simulink model "Control_Logic_b_chk2"  (R2019b)
settings: Solver=VariableStepAuto  StartTime=Start_time  StopTime=Stop_time  RelTol=1e-3
values from neighbouring files (symbols this model uses):
  Aset_N1 = 2    [Parameter_control.m]
  Aset_N10 = -10    [Parameter_control.m]
  Aset_N11 = 10    [Parameter_control.m]
  Aset_N12 = 20    [Parameter_control.m]
  Aset_N2 = 30    [Parameter_control.m]
  Aset_N3 = 3    [Parameter_control.m]
  Aset_N4 = 5    [Parameter_control.m]
  Aset_N5 = 1    [Parameter_control.m]
  Aset_N6 = 0    [Parameter_control.m]
  Aset_N7 = 0.01    [Parameter_control.m]
  Aset_N8 = 2    [Parameter_control.m]
  Aset_N9 = 0.1    [Parameter_control.m]
  Dset_N1 = 1    [Parameter_control.m]
  Dset_N2 = 1    [Parameter_control.m]
  Sample_time = 0.1    [main.m]    (also in test_tool_initialize.m)
undefined symbols (not defined in the file or in its folder): DiscIntNeverNeededParam
(part 1 of 3)
settings Model: Creator=M156732  LastModifiedBy=yangy
settings DataIOCC: ReturnWorkspaceOutputs=off
settings DebuggingCC: ArithmeticOperatorsInVariantConditions=warning
settings ModelReferenceCC: ModelReferenceNumInstancesAllowed=Single
settings SFSimCC: CustomCodeUndefinedFunction=UseInterfaceOnly

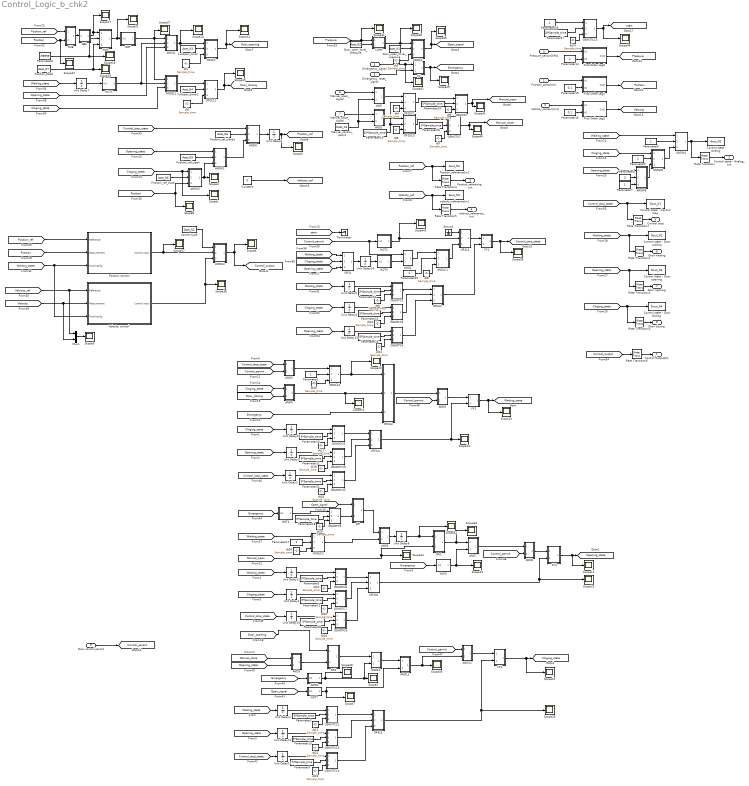
== system Control_Logic_b_chk2 ==
  Position_sensor[m] : Inport  OutDataTypeStr=double  Unit=mm  SampleTime=Sample_time
  Velocity_sensor[m/s] : Inport  Port=2  OutDataTypeStr=double  Unit=mm  SampleTime=Sample_time
  Pressure_sensor[kPa] : Inport  Port=3  OutDataTypeStr=double  Unit=kPa  SampleTime=Sample_time
  Emergency_signal : Inport  Port=4  OutDataTypeStr=boolean  SampleTime=Sample_time
  Emergency_reset_signal : Inport  Port=5  OutDataTypeStr=boolean  SampleTime=Sample_time
  Manual_open_signal : Inport  Port=6  OutDataTypeStr=boolean  SampleTime=Sample_time
  Manual_close_signal : Inport  Port=7  OutDataTypeStr=boolean  SampleTime=Sample_time
  Door control permit : Inport  Port=8  OutDataTypeStr=boolean  SampleTime=Sample_time
  ABS : Subsystem
  AND : Subsystem
  AND1 : Subsystem
  AND10 : Subsystem
  AND11 : Subsystem
  AND12 : Subsystem
  AND2 : Subsystem
  AND3 : Subsystem
  AND3L : Subsystem
  AND3L1 : Subsystem
  AND4 : Subsystem
  AND5 : Subsystem
  AND6 : Subsystem
  AND7 : Subsystem
  AND8 : Subsystem
  AND9 : Subsystem
  ANSW : Subsystem
  ANSW1 : Subsystem
  ANSW2 : Subsystem
  ANSW3 : Subsystem
  ANSW4 : Subsystem
  ANSW5 : Subsystem
  ANSW6 : Subsystem
  COMP : Subsystem
  Constant : Constant  Value=0
  Control state - Analog : ToWorkspace  VariableName=Aout_N2  SampleTime=Sample_time
  Control state - Control stop : ToWorkspace  VariableName=Dout_N1  SampleTime=Sample_time
  Control state - Door closing : ToWorkspace  VariableName=Dout_N4  SampleTime=Sample_time
  Control state - Door opening : ToWorkspace  VariableName=Dout_N3  SampleTime=Sample_time
  Control state - Door waiting : ToWorkspace  VariableName=Dout_N2  SampleTime=Sample_time
  Door_open_level_pressure : Constant  Value=Aset_N2  OutDataTypeStr=double  SampleTime=Sample_time
  Door_open_timer_pressure : Constant  Value=Aset_N1  OutDataTypeStr=double  SampleTime=Sample_time
  FF : Subsystem
  FF1 : Subsystem
  FF2 : Subsystem
  FF3 : Subsystem
  FF4 : Subsystem
  First Order Lag1 : Subsystem
  First Order Lag2 : Subsystem
  First Order Lag5 : Subsystem
  Fullopen_timer : Constant  Value=Aset_N3  OutDataTypeStr=double  SampleTime=Sample_time
  Fullopen_timer1 : Constant  Value=Aset_N4  OutDataTypeStr=double  SampleTime=Sample_time
  Ground : Ground
  HLM : Subsystem
  Manual_control_pemit : Constant  Value=Dset_N1  OutDataTypeStr=boolean  SampleTime=Sample_time
  Mux1 : Mux  Inputs=2
  NOT : Subsystem
  NOT1 : Subsystem
  NOT2 : Subsystem
  NOT3 : Subsystem
  NOT4 : Subsystem
  NOT5 : Subsystem
  NOT6 : Subsystem
  NOT7 : Subsystem
  OFDLC : Subsystem
  OFDLC1 : Subsystem
  OFDLC2 : Subsystem
  OFDLC3 : Subsystem
  ONDLC : Subsystem
  ONDLC1 : Subsystem
  ONDLC2 : Subsystem
  ONDLC3 : Subsystem
  OR : Subsystem
  OR1 : Subsystem
  OR2 : Subsystem
  OR3L : Subsystem
  OR3L1 : Subsystem
  OR3L2 : Subsystem
  OR3L3 : Subsystem
  OR3L4 : Subsystem
  OR3L5 : Subsystem
  OR3L6 : Subsystem
  OSHOTC : Subsystem
  OSHOTC1 : Subsystem
  OSHOTC10 : Subsystem
  OSHOTC11 : Subsystem
  OSHOTC12 : Subsystem
  OSHOTC13 : Subsystem
  OSHOTC14 : Subsystem
  OSHOTC15 : Subsystem
  OSHOTC2 : Subsystem
  OSHOTC3 : Subsystem
  OSHOTC4 : Subsystem
  OSHOTC5 : Subsystem
  OSHOTC6 : Subsystem
  OSHOTC7 : Subsystem
  OSHOTC8 : Subsystem
  OSHOTC9 : Subsystem
  Parameter{1,6..7,25} (4 alike) : Constant  OutDataTypeStr=int32  SampleTime=Sample_time
  Parameter{2..3,9..13,18,20..24,28..29} (15 alike) : Constant  Value=5*Sample_time  OutDataTypeStr=double  SampleTime=Sample_time
  Parameter14 : Constant  OutDataTypeStr=double  SampleTime=Sample_time
  Parameter15 : Constant  Value=0.1  OutDataTypeStr=double  SampleTime=Sample_time
  Parameter16 : Constant  Value=0.1  OutDataTypeStr=double  SampleTime=Sample_time
  Parameter17 : Constant  Value=2  OutDataTypeStr=int32  SampleTime=Sample_time
  Parameter19 : Constant  Value=10*Sample_time  OutDataTypeStr=double  SampleTime=Sample_time
  Parameter26 : Constant  OutDataTypeStr=boolean  SampleTime=Sample_time
  Parameter27 : Constant  Value=10*Sample_time  OutDataTypeStr=double  SampleTime=Sample_time
  Parameter4 : Constant  Value=3  OutDataTypeStr=int32  SampleTime=Sample_time
  Parameter5 : Constant  Value=2  OutDataTypeStr=int32  SampleTime=Sample_time
  Parameter8 : Constant  Value=-99999  OutDataTypeStr=double  SampleTime=Sample_time
  Position control : Subsystem
  Position_delta : Constant  Value=Aset_N7  OutDataTypeStr=double  SampleTime=Sample_time
  Position_ref_close : Constant  Value=Aset_N6  OutDataTypeStr=double  SampleTime=Sample_time
  Position_ref_close1 : Constant  Value=Aset_N6  OutDataTypeStr=double  SampleTime=Sample_time
  Position_ref_open : Constant  Value=Aset_N5  OutDataTypeStr=double  SampleTime=Sample_time
  Position_reference[m] : ToWorkspace  VariableName=Aout_N3  SampleTime=Sample_time
  Rate Transition{,1..7} (8 alike) : RateTransition  OutPortSampleTime=Sample_time
  SUB : Subsystem
  Scope{1..4,6..44} (43 alike) : Scope
  Terminator : Terminator
  Unit Delay{1..13,15..16} (15 alike) : UnitDelay  SampleTime=Sample_time  HasFrameUpgradeWarning=on
  Unit Delay14 : UnitDelay  InitialCondition=1  SampleTime=Sample_time  HasFrameUpgradeWarning=on
  Velocity control : Subsystem
  control type : Constant  Value=Dset_N2  OutDataTypeStr=boolean  SampleTime=Sample_time
  dt{1..12,14..19,21..24} (22 alike) : Constant  Value=Sample_time  OutDataTypeStr=double  SampleTime=Sample_time
  dt25 : Constant  Value=Sample_time  OutDataTypeStr=double
  dt26 : Constant  Value=Sample_time  OutDataTypeStr=double
  velocity_reference[m] : ToWorkspace  VariableName=Aout_N4  SampleTime=Sample_time
  Control Output[N] : Outport  OutDataTypeStr=double  Unit=N  SampleTime=Sample_time  VectorParamsAs1DForOutWhenUnconnected=off  LockScale=on
  Control state - Analog_out : Outport  Port=2  SampleTime=Sample_time  VectorParamsAs1DForOutWhenUnconnected=off
  Position_reference_out : Outport  Port=3  SampleTime=Sample_time  VectorParamsAs1DForOutWhenUnconnected=off
  velocity_reference_out : Outport  Port=4  SampleTime=Sample_time  VectorParamsAs1DForOutWhenUnconnected=off
  Control stop : Outport  Port=5  SampleTime=Sample_time  VectorParamsAs1DForOutWhenUnconnected=off
  Door waiting : Outport  Port=6  SampleTime=Sample_time  VectorParamsAs1DForOutWhenUnconnected=off
  Door opening : Outport  Port=7  SampleTime=Sample_time  VectorParamsAs1DForOutWhenUnconnected=off
  Door closing : Outport  Port=8  SampleTime=Sample_time  VectorParamsAs1DForOutWhenUnconnected=off
  tag scope: Cloging_state=global, Control_output=global, Control_permit=global, Control_stop_state=global, Door_closing=global, Door_opening=global, Emergency=global, Manual_close=global, Manual_open=global, Open_signal=global, Opening_state=global, Position=global, Position_ref=global, Pressure=global, Velocity=global, Velocity_ref=global, Waiting_state=global, start=global
  wires:
  FF2/1(Out1) -> Scope10/1, [Waiting_state]
  FF3/1(Out1) -> [Cloging_state], Scope12/1
  FF4/1(Out1) -> [Opening_state], Scope11/1
  AND4/1(Out1) -> Scope16/1, OR3L3/2(In2)
  [Emergency] -> OR3L3/3(In3)
  [Door_closing] -> AND4/2(In2)
  [Cloging_state] -> AND4/1(In1)
  [Manual_open] -> OR1/2(In2), Scope34/1
  OR1/1(Out1) -> AND7/1(In1), Scope33/1
  [Door_opening] -> OR2/1(In1)
  Door_open_timer_pressure/1 -> ONDLC/2(In2)
  Door_open_level_pressure/1 -> COMP/2(In2)
  COMP/1(Out1) -> ONDLC/1(In1), Scope30/1
  ONDLC/1(Out1) -> Scope35/1, [Open_signal]
  FF/1(Out1) -> Scope29/1, [Emergency]
  Emergency_reset_signal/1 -> FF/2(In2)
  ANSW5/1(Out1) -> ANSW4/3(In3)
  ANSW6/1(Out1) -> ANSW5/3(In3)
  Parameter4/1 -> ANSW6/2(In2)
  Parameter5/1 -> ANSW5/2(In2)
  Parameter6/1 -> ANSW4/2(In2)
  Parameter7/1 -> ANSW6/3(In3)
  ANSW4/1(Out1) -> Rate Transition/1, Control state - Analog/1
  Manual_control_pemit/1 -> AND1/2(In2), AND/2(In2)
  [Position_ref] -> SUB/1(In1)
  SUB/1(Out1) -> ABS/1(In1)
  Position_delta/1 -> HLM/3(In3), Scope19/1
  Parameter8/1 -> HLM/2(In2), Scope18/1
  HLM/1(Out1) -> NOT/1(In1), Scope21/1
  Fullopen_timer/1 -> OFDLC/2(In2)
  [Opening_state] -> ANSW1/1(In1)
  ANSW2/1(Out1) -> Scope4/1, ANSW1/3(In3)
  [Cloging_state] -> Scope1/1, ANSW2/1(In1)
  Position_ref_open/1 -> ANSW1/2(In2)
  Position_ref_close/1 -> ANSW2/2(In2)
  [Position] -> ANSW2/3(In3), Scope8/1
  Fullopen_timer1/1 -> OFDLC1/2(In2)
  [Waiting_state] -> Rate Transition1/1, Control state - Door waiting/1
  [Opening_state] -> Rate Transition2/1, Control state - Door opening/1
  [Cloging_state] -> Rate Transition3/1, Control state - Door closing/1
  [Position] -> Scope22/1, SUB/2(In2)
  Unit Delay6/1 -> Scope3/1, [Position_ref]
  [Pressure] -> COMP/1(In1), Scope31/1
  Parameter1/1 -> ONDLC2/2(In2)
  AND3/1(Out1) -> ONDLC2/1(In1)
  ONDLC2/1(Out1) -> Scope23/1, OR3L3/1(In1)
  ABS/1(Out1) -> HLM/1(In1), Scope17/1
  OFDLC/1(Out1) -> Scope14/1, [Door_opening]
  OFDLC1/1(Out1) -> Scope15/1, [Door_closing]
  [Waiting_state] -> Unit Delay7/1
  NOT/1(Out1) -> AND3L1/1(In1), AND3L/1(In1), Scope27/1
  AND3L/1(Out1) -> OFDLC/1(In1), Scope20/1
  NOT1/1(Out1) -> AND3L1/2(In2), AND3L/2(In2)
  Unit Delay7/1 -> NOT1/1(In1)
  OR3L4/1(Out1) -> FF2/2(In2), Scope24/1
  AND6/1(Out1) -> Unit Delay8/1
  Unit Delay8/1 -> OR1/1(In1), Scope32/1
  [Opening_state] -> AND3L/3(In3)
  [Cloging_state] -> AND3L1/3(In3)
  AND3L1/1(Out1) -> OFDLC1/1(In1)
  [Opening_state] -> Unit Delay1/1
  [Cloging_state] -> Unit Delay10/1
  Parameter10/1 -> OSHOTC9/2(In2)
  OSHOTC9/1(Out1) -> OR3L4/1(In1)
  Unit Delay10/1 -> OSHOTC9/1(In1)
  Unit Delay1/1 -> OSHOTC10/1(In1)
  Parameter11/1 -> OSHOTC10/2(In2)
  OSHOTC10/1(Out1) -> OR3L4/2(In2)
  Parameter12/1 -> OSHOTC7/2(In2)
  OR3L6/1(Out1) -> FF4/2(In2), Scope25/1
  OSHOTC7/1(Out1) -> OR3L6/2(In2)
  Parameter3/1 -> OSHOTC6/2(In2)
  [Waiting_state] -> Unit Delay11/1
  OSHOTC6/1(Out1) -> OR3L6/1(In1)
  Unit Delay11/1 -> OSHOTC6/1(In1)
  [Cloging_state] -> Unit Delay4/1
  Unit Delay4/1 -> OSHOTC7/1(In1)
  [Waiting_state] -> Unit Delay2/1
  Parameter2/1 -> OSHOTC12/2(In2)
  OR3L5/1(Out1) -> FF3/2(In2), Scope26/1
  OSHOTC12/1(Out1) -> OR3L5/1(In1)
  Parameter13/1 -> OSHOTC13/2(In2)
  [Opening_state] -> Unit Delay12/1
  OSHOTC13/1(Out1) -> OR3L5/2(In2)
  Unit Delay2/1 -> OSHOTC12/1(In1)
  Unit Delay12/1 -> OSHOTC13/1(In1)
  [Position_ref] -> Position control/1(Reference)
  [Position] -> Position control/2(Measurement)
  [Waiting_state] -> Velocity control/3(Tracking flg), Position control/3(Tracking flg)
  Position control/1(Control input) -> ANSW3/2(In2), Scope37/1
  ANSW3/1(Out1) -> [Control_output], Scope6/1
  Velocity control/1(Control input) -> ANSW3/3(In3), Scope38/1
  control type/1 -> ANSW3/1(In1)
  [Velocity] -> Velocity control/2(Measurement), Mux1/2
  [Velocity_ref] -> Velocity control/1(Reference), Mux1/1
  Mux1/1 -> Scope9/1
  Pressure_sensor[kPa]/1 -> First Order Lag5/1(In1)
  First Order Lag5/1(Out1) -> [Pressure]
  First Order Lag1/1(Out1) -> [Position]
  Position_sensor[m]/1 -> First Order Lag1/1(In1)
  First Order Lag2/1(Out1) -> [Velocity]
  Velocity_sensor[m/s]/1 -> First Order Lag2/1(In1)
  Parameter14/1 -> First Order Lag5/2(In2)
  Parameter15/1 -> First Order Lag1/2(In2)
  Parameter16/1 -> First Order Lag2/2(In2)
  [Waiting_state] -> ANSW4/1(In1)
  [Cloging_state] -> ANSW5/1(In1)
  [Opening_state] -> ANSW6/1(In1)
  Rate Transition/1 -> Control state - Analog_out/1
  Rate Transition1/1 -> Door waiting/1
  Rate Transition2/1 -> Door opening/1
  Rate Transition3/1 -> Door closing/1
  Parameter17/1 -> ONDLC3/2(In2)
  [Waiting_state] -> ONDLC3/1(In1)
  ONDLC3/1(Out1) -> AND6/2(In2)
  [Position_ref] -> Rate Transition4/1, Position_reference[m]/1
  Rate Transition4/1 -> Position_reference_out/1
  Rate Transition5/1 -> velocity_reference_out/1
  [Velocity_ref] -> velocity_reference[m]/1, Rate Transition5/1
  [Emergency] -> NOT5/1(In1)
  NOT5/1(Out1) -> AND7/2(In2), Scope13/1
  [Emergency] -> NOT6/1(In1)
  OR2/1(Out1) -> AND10/1(In1)
  OR/1(Out1) -> AND6/1(In1)
  [Open_signal] -> OR/1(In1)
  [Emergency] -> NOT4/1(In1)
  Parameter18/1 -> OSHOTC5/2(In2)
  OSHOTC5/1(Out1) -> OR/2(In2)
  NOT4/1(Out1) -> OSHOTC5/1(In1)
  Manual_open_signal/1 -> AND/1(In1)
  Manual_close_signal/1 -> AND1/1(In1)
  AND1/1(Out1) -> OFDLC3/1(In1)
  AND/1(Out1) -> OFDLC2/1(In1)
  Parameter19/1 -> OFDLC3/2(In2), OFDLC2/2(In2)
  AND9/1(Out1) -> OR2/2(In2)
  [Opening_state] -> AND9/2(In2)
  [Open_signal] -> NOT7/1(In1)
  NOT7/1(Out1) -> Scope7/1, AND11/2(In2)
  NOT6/1(Out1) -> Scope28/1, AND10/2(In2), Scope2/1
  Emergency_signal/1 -> FF/1(In1), Scope42/1
  AND10/1(Out1) -> AND11/1(In1)
  OSHOTC14/1(Out1) -> OR3L5/3(In3)
  Door control permit/1 -> [Control_permit]
  OSHOTC8/1(Out1) -> OR3L6/3(In3)
  OSHOTC11/1(Out1) -> OR3L4/3(In3)
  AND12/1(Out1) -> FF3/1(In1)
  AND11/1(Out1) -> AND12/2(In2), Scope39/1
  [Control_permit] -> AND12/1(In1)
  AND7/1(Out1) -> AND8/1(In1)
  AND8/1(Out1) -> FF4/1(In1)
  [Control_permit] -> AND8/2(In2)
  [Control_permit] -> AND5/2(In2)
  OR3L3/1(Out1) -> AND5/1(In1)
  AND5/1(Out1) -> FF2/1(In1)
  FF1/1(Out1) -> Scope36/1, [Control_stop_state]
  [Control_permit] -> AND2/1(In1), NOT2/1(In1)
  OSHOTC4/1(Out1) -> OR3L2/3(In3)
  Unit Delay9/1 -> OSHOTC3/1(In1)
  [Cloging_state] -> Unit Delay9/1
  Unit Delay5/1 -> OSHOTC2/1(In1)
  OSHOTC2/1(Out1) -> OR3L2/1(In1)
  [Waiting_state] -> Unit Delay5/1
  Parameter23/1 -> OSHOTC2/2(In2)
  OSHOTC3/1(Out1) -> OR3L2/2(In2)
  Parameter22/1 -> OSHOTC3/2(In2)
  Parameter24/1 -> OSHOTC4/2(In2)
  Unit Delay13/1 -> OSHOTC4/1(In1)
  [Opening_state] -> Unit Delay13/1
  OR3L2/1(Out1) -> FF1/2(In2)
  Rate Transition6/1 -> Control Output[N]/1
  [Control_output] -> Rate Transition6/1
  Rate Transition7/1 -> Control stop/1
  [Control_stop_state] -> Control state - Control stop/1, Rate Transition7/1
  Constant/1 -> [Velocity_ref]
  NOT2/1(Out1) -> OR3L1/2(In2), Scope43/1
  OR3L1/1(Out1) -> FF1/1(In1)
  [Cloging_state] -> OR3L/2(In2)
  Unit Delay14/1 -> NOT3/1(In1)
  [Waiting_state] -> OR3L/1(In1)
  OR3L/1(Out1) -> Unit Delay14/1
  [Opening_state] -> OR3L/3(In3)
  Parameter25/1 -> ONDLC1/2(In2)
  [Control_stop_state] -> AND3/1(In1)
  [Control_permit] -> AND3/2(In2)
  Parameter26/1 -> OSHOTC15/1(In1)
  OSHOTC15/1(Out1) -> Scope44/1, [start]
  Parameter27/1 -> OSHOTC15/2(In2)
  AND2/1(Out1) -> ONDLC1/1(In1)
  NOT3/1(Out1) -> AND2/2(In2)
  ONDLC1/1(Out1) -> OR3L1/3(In3)
  Parameter21/1 -> OSHOTC11/2(In2)
  Unit Delay3/1 -> OSHOTC11/1(In1)
  [Control_stop_state] -> Unit Delay3/1
  [Control_stop_state] -> Unit Delay15/1
  Unit Delay15/1 -> OSHOTC8/1(In1)
  Parameter20/1 -> OSHOTC8/2(In2)
  Parameter9/1 -> OSHOTC14/2(In2)
  Unit Delay16/1 -> OSHOTC14/1(In1)
  [Control_stop_state] -> Unit Delay16/1
  ANSW1/1(Out1) -> ANSW/3(In3)
  ANSW/1(Out1) -> Unit Delay6/1
  [Control_stop_state] -> ANSW/1(In1)
  Position_ref_close1/1 -> ANSW/2(In2)
  [Manual_close] -> AND9/1(In1)
  Parameter28/1 -> OSHOTC1/2(In2)
  OFDLC3/1(Out1) -> OSHOTC1/1(In1)
  OFDLC2/1(Out1) -> OSHOTC/1(In1)
  Parameter29/1 -> OSHOTC/2(In2)
  OSHOTC/1(Out1) -> [Manual_open], Scope41/1
  OSHOTC1/1(Out1) -> [Manual_close], Scope40/1
  Ground/1 -> OR3L1/1(In1)
  [start] -> Terminator/1
  dt1/1 -> OFDLC/3(In3)
  dt2/1 -> OFDLC1/3(In3)
  dt3/1 -> ONDLC/3(In3)
  dt4/1 -> OFDLC2/3(In3)
  dt5/1 -> OFDLC3/3(In3)
  dt6/1 -> OSHOTC/3(In3)
  dt7/1 -> OSHOTC1/3(In3)
  dt8/1 -> ONDLC1/3(In3)
  dt9/1 -> OSHOTC2/3(In3)
  dt10/1 -> OSHOTC3/3(In3)
  dt11/1 -> OSHOTC4/3(In3)
  dt12/1 -> ONDLC2/3(In3)
  dt25/1 -> OSHOTC5/3(In3)
  dt14/1 -> OSHOTC6/3(In3)
  dt15/1 -> OSHOTC7/3(In3)
  dt16/1 -> OSHOTC8/3(In3)
  dt17/1 -> OSHOTC9/3(In3)
  dt18/1 -> OSHOTC10/3(In3)
  dt19/1 -> OSHOTC11/3(In3)
  dt26/1 -> ONDLC3/3(In3)
  dt21/1 -> OSHOTC12/3(In3)
  dt22/1 -> OSHOTC13/3(In3)
  dt23/1 -> OSHOTC14/3(In3)
  dt24/1 -> OSHOTC15/3(In3)

== system Control_Logic_b_chk2/ABS ==
  In1 : Inport
  MATLAB Function : MATLAB Function  TreatAsAtomicUnit=on  SystemSampleTime=Sample_time
  Out1 : Outport  VectorParamsAs1DForOutWhenUnconnected=off
  wires:
  In1/1 -> MATLAB Function/1(u)
  MATLAB Function/1(y) -> Out1/1

== system Control_Logic_b_chk2/AND ==
  In1 : Inport
  In2 : Inport  Port=2
  MATLAB Function : MATLAB Function  TreatAsAtomicUnit=on  SystemSampleTime=Sample_time
  Mux : Mux  Inputs=2
  Out1 : Outport  VectorParamsAs1DForOutWhenUnconnected=off
  wires:
  Mux/1 -> MATLAB Function/1(u)
  In2/1 -> Mux/2
  MATLAB Function/1(y) -> Out1/1
  In1/1 -> Mux/1

== system Control_Logic_b_chk2/AND1 ==
  In1 : Inport
  In2 : Inport  Port=2
  MATLAB Function : MATLAB Function  TreatAsAtomicUnit=on  SystemSampleTime=Sample_time
  Mux : Mux  Inputs=2
  Out1 : Outport  VectorParamsAs1DForOutWhenUnconnected=off
  wires:
  Mux/1 -> MATLAB Function/1(u)
  In2/1 -> Mux/2
  MATLAB Function/1(y) -> Out1/1
  In1/1 -> Mux/1

== system Control_Logic_b_chk2/AND10 ==
  In1 : Inport
  In2 : Inport  Port=2
  MATLAB Function : MATLAB Function  TreatAsAtomicUnit=on  SystemSampleTime=Sample_time
  Mux : Mux  Inputs=2
  Out1 : Outport  VectorParamsAs1DForOutWhenUnconnected=off
  wires:
  Mux/1 -> MATLAB Function/1(u)
  In2/1 -> Mux/2
  MATLAB Function/1(y) -> Out1/1
  In1/1 -> Mux/1

== system Control_Logic_b_chk2/AND11 ==
  In1 : Inport
  In2 : Inport  Port=2
  MATLAB Function : MATLAB Function  TreatAsAtomicUnit=on  SystemSampleTime=Sample_time
  Mux : Mux  Inputs=2
  Out1 : Outport  VectorParamsAs1DForOutWhenUnconnected=off
  wires:
  Mux/1 -> MATLAB Function/1(u)
  In2/1 -> Mux/2
  MATLAB Function/1(y) -> Out1/1
  In1/1 -> Mux/1

== system Control_Logic_b_chk2/AND12 ==
  In1 : Inport
  In2 : Inport  Port=2
  MATLAB Function : MATLAB Function  TreatAsAtomicUnit=on  SystemSampleTime=Sample_time
  Mux : Mux  Inputs=2
  Out1 : Outport  VectorParamsAs1DForOutWhenUnconnected=off
  wires:
  Mux/1 -> MATLAB Function/1(u)
  In2/1 -> Mux/2
  MATLAB Function/1(y) -> Out1/1
  In1/1 -> Mux/1

== system Control_Logic_b_chk2/AND2 ==
  In1 : Inport
  In2 : Inport  Port=2
  MATLAB Function : MATLAB Function  TreatAsAtomicUnit=on  SystemSampleTime=Sample_time
  Mux : Mux  Inputs=2
  Out1 : Outport  VectorParamsAs1DForOutWhenUnconnected=off
  wires:
  Mux/1 -> MATLAB Function/1(u)
  In2/1 -> Mux/2
  MATLAB Function/1(y) -> Out1/1
  In1/1 -> Mux/1

== system Control_Logic_b_chk2/AND3 ==
  In1 : Inport
  In2 : Inport  Port=2
  MATLAB Function : MATLAB Function  TreatAsAtomicUnit=on  SystemSampleTime=Sample_time
  Mux : Mux  Inputs=2
  Out1 : Outport  VectorParamsAs1DForOutWhenUnconnected=off
  wires:
  Mux/1 -> MATLAB Function/1(u)
  In2/1 -> Mux/2
  MATLAB Function/1(y) -> Out1/1
  In1/1 -> Mux/1

== system Control_Logic_b_chk2/AND3L ==
  In1 : Inport
  In2 : Inport  Port=2
  In3 : Inport  Port=3
  MATLAB Function : MATLAB Function  TreatAsAtomicUnit=on  SystemSampleTime=Sample_time
  Mux : Mux  Inputs=3
  Out1 : Outport  VectorParamsAs1DForOutWhenUnconnected=off
  wires:
  MATLAB Function/1(y) -> Out1/1
  Mux/1 -> MATLAB Function/1(u)
  In2/1 -> Mux/3
  In3/1 -> Mux/2
  In1/1 -> Mux/1

== system Control_Logic_b_chk2/AND3L1 ==
  In1 : Inport
  In2 : Inport  Port=2
  In3 : Inport  Port=3
  MATLAB Function : MATLAB Function  TreatAsAtomicUnit=on  SystemSampleTime=Sample_time
  Mux : Mux  Inputs=3
  Out1 : Outport  VectorParamsAs1DForOutWhenUnconnected=off
  wires:
  MATLAB Function/1(y) -> Out1/1
  Mux/1 -> MATLAB Function/1(u)
  In2/1 -> Mux/3
  In3/1 -> Mux/2
  In1/1 -> Mux/1

== system Control_Logic_b_chk2/AND4 ==
  In1 : Inport
  In2 : Inport  Port=2
  MATLAB Function : MATLAB Function  TreatAsAtomicUnit=on  SystemSampleTime=Sample_time
  Mux : Mux  Inputs=2
  Out1 : Outport  VectorParamsAs1DForOutWhenUnconnected=off
  wires:
  Mux/1 -> MATLAB Function/1(u)
  In2/1 -> Mux/2
  MATLAB Function/1(y) -> Out1/1
  In1/1 -> Mux/1

== system Control_Logic_b_chk2/AND5 ==
  In1 : Inport
  In2 : Inport  Port=2
  MATLAB Function : MATLAB Function  TreatAsAtomicUnit=on  SystemSampleTime=Sample_time
  Mux : Mux  Inputs=2
  Out1 : Outport  VectorParamsAs1DForOutWhenUnconnected=off
  wires:
  Mux/1 -> MATLAB Function/1(u)
  In2/1 -> Mux/2
  MATLAB Function/1(y) -> Out1/1
  In1/1 -> Mux/1

== system Control_Logic_b_chk2/AND6 ==
  In1 : Inport
  In2 : Inport  Port=2
  MATLAB Function : MATLAB Function  TreatAsAtomicUnit=on  SystemSampleTime=Sample_time
  Mux : Mux  Inputs=2
  Out1 : Outport  VectorParamsAs1DForOutWhenUnconnected=off
  wires:
  Mux/1 -> MATLAB Function/1(u)
  In2/1 -> Mux/2
  MATLAB Function/1(y) -> Out1/1
  In1/1 -> Mux/1

== system Control_Logic_b_chk2/AND7 ==
  In1 : Inport
  In2 : Inport  Port=2
  MATLAB Function : MATLAB Function  TreatAsAtomicUnit=on  SystemSampleTime=Sample_time
  Mux : Mux  Inputs=2
  Out1 : Outport  VectorParamsAs1DForOutWhenUnconnected=off
  wires:
  Mux/1 -> MATLAB Function/1(u)
  In2/1 -> Mux/2
  MATLAB Function/1(y) -> Out1/1
  In1/1 -> Mux/1

== system Control_Logic_b_chk2/AND8 ==
  In1 : Inport
  In2 : Inport  Port=2
  MATLAB Function : MATLAB Function  TreatAsAtomicUnit=on  SystemSampleTime=Sample_time
  Mux : Mux  Inputs=2
  Out1 : Outport  VectorParamsAs1DForOutWhenUnconnected=off
  wires:
  Mux/1 -> MATLAB Function/1(u)
  In2/1 -> Mux/2
  MATLAB Function/1(y) -> Out1/1
  In1/1 -> Mux/1

== system Control_Logic_b_chk2/AND9 ==
  In1 : Inport
  In2 : Inport  Port=2
  MATLAB Function : MATLAB Function  TreatAsAtomicUnit=on  SystemSampleTime=Sample_time
  Mux : Mux  Inputs=2
  Out1 : Outport  VectorParamsAs1DForOutWhenUnconnected=off
  wires:
  Mux/1 -> MATLAB Function/1(u)
  In2/1 -> Mux/2
  MATLAB Function/1(y) -> Out1/1
  In1/1 -> Mux/1

== system Control_Logic_b_chk2/ANSW ==
  In1 : Inport
  In2 : Inport  Port=2
  In3 : Inport  Port=3
  MATLAB Function : MATLAB Function  TreatAsAtomicUnit=on  SystemSampleTime=Sample_time
  Mux : Mux  Inputs=2
  Out1 : Outport  VectorParamsAs1DForOutWhenUnconnected=off
  wires:
  In1/1 -> MATLAB Function/1(ud)
  Mux/1 -> MATLAB Function/2(ua)
  MATLAB Function/1(y) -> Out1/1
  In3/1 -> Mux/2
  In2/1 -> Mux/1

== system Control_Logic_b_chk2/ANSW1 ==
  In1 : Inport
  In2 : Inport  Port=2
  In3 : Inport  Port=3
  MATLAB Function : MATLAB Function  TreatAsAtomicUnit=on  SystemSampleTime=Sample_time
  Mux : Mux  Inputs=2
  Out1 : Outport  VectorParamsAs1DForOutWhenUnconnected=off
  wires:
  In1/1 -> MATLAB Function/1(ud)
  Mux/1 -> MATLAB Function/2(ua)
  MATLAB Function/1(y) -> Out1/1
  In3/1 -> Mux/2
  In2/1 -> Mux/1

== system Control_Logic_b_chk2/ANSW2 ==
  In1 : Inport
  In2 : Inport  Port=2
  In3 : Inport  Port=3
  MATLAB Function : MATLAB Function  TreatAsAtomicUnit=on  SystemSampleTime=Sample_time
  Mux : Mux  Inputs=2
  Out1 : Outport  VectorParamsAs1DForOutWhenUnconnected=off
  wires:
  In1/1 -> MATLAB Function/1(ud)
  Mux/1 -> MATLAB Function/2(ua)
  MATLAB Function/1(y) -> Out1/1
  In3/1 -> Mux/2
  In2/1 -> Mux/1

== system Control_Logic_b_chk2/ANSW3 ==
  In1 : Inport
  In2 : Inport  Port=2
  In3 : Inport  Port=3
  MATLAB Function : MATLAB Function  TreatAsAtomicUnit=on  SystemSampleTime=Sample_time
  Mux : Mux  Inputs=2
  Out1 : Outport  VectorParamsAs1DForOutWhenUnconnected=off
  wires:
  In1/1 -> MATLAB Function/1(ud)
  Mux/1 -> MATLAB Function/2(ua)
  MATLAB Function/1(y) -> Out1/1
  In3/1 -> Mux/2
  In2/1 -> Mux/1

== system Control_Logic_b_chk2/ANSW4 ==
  In1 : Inport
  In2 : Inport  Port=2
  In3 : Inport  Port=3
  MATLAB Function : MATLAB Function  TreatAsAtomicUnit=on  SystemSampleTime=Sample_time
  Mux : Mux  Inputs=2
  Out1 : Outport  VectorParamsAs1DForOutWhenUnconnected=off
  wires:
  In1/1 -> MATLAB Function/1(ud)
  Mux/1 -> MATLAB Function/2(ua)
  MATLAB Function/1(y) -> Out1/1
  In3/1 -> Mux/2
  In2/1 -> Mux/1

== system Control_Logic_b_chk2/ANSW5 ==
  In1 : Inport
  In2 : Inport  Port=2
  In3 : Inport  Port=3
  MATLAB Function : MATLAB Function  TreatAsAtomicUnit=on  SystemSampleTime=Sample_time
  Mux : Mux  Inputs=2
  Out1 : Outport  VectorParamsAs1DForOutWhenUnconnected=off
  wires:
  In1/1 -> MATLAB Function/1(ud)
  Mux/1 -> MATLAB Function/2(ua)
  MATLAB Function/1(y) -> Out1/1
  In3/1 -> Mux/2
  In2/1 -> Mux/1

== system Control_Logic_b_chk2/ANSW6 ==
  In1 : Inport
  In2 : Inport  Port=2
  In3 : Inport  Port=3
  MATLAB Function : MATLAB Function  TreatAsAtomicUnit=on  SystemSampleTime=Sample_time
  Mux : Mux  Inputs=2
  Out1 : Outport  VectorParamsAs1DForOutWhenUnconnected=off
  wires:
  In1/1 -> MATLAB Function/1(ud)
  Mux/1 -> MATLAB Function/2(ua)
  MATLAB Function/1(y) -> Out1/1
  In3/1 -> Mux/2
  In2/1 -> Mux/1

== system Control_Logic_b_chk2/COMP ==
  In1 : Inport
  In2 : Inport  Port=2
  MATLAB Function : MATLAB Function  TreatAsAtomicUnit=on  SystemSampleTime=Sample_time
  Out1 : Outport  VectorParamsAs1DForOutWhenUnconnected=off
  wires:
  In2/1 -> MATLAB Function/2(set)
  MATLAB Function/1(y) -> Out1/1
  In1/1 -> MATLAB Function/1(u)

== system Control_Logic_b_chk2/FF ==
  In1 : Inport
  In2 : Inport  Port=2
  Data Type Conversion : DataTypeConversion  OutDataTypeStr=boolean
  MATLAB Function : MATLAB Function  TreatAsAtomicUnit=on  SystemSampleTime=Sample_time
  Memory : Memory  InheritSampleTime=on
  Mux : Mux  Inputs=2
  Out1 : Outport  VectorParamsAs1DForOutWhenUnconnected=off
  wires:
  Mux/1 -> MATLAB Function/2(set)
  Memory/1 -> Data Type Conversion/1
  In1/1 -> Mux/1
  MATLAB Function/1(y) -> Out1/1, Memory/1
  Data Type Conversion/1 -> MATLAB Function/1(yold)
  In2/1 -> Mux/2

== system Control_Logic_b_chk2/FF1 ==
  In1 : Inport
  In2 : Inport  Port=2
  Data Type Conversion : DataTypeConversion  OutDataTypeStr=boolean
  MATLAB Function : MATLAB Function  TreatAsAtomicUnit=on  SystemSampleTime=Sample_time
  Memory : Memory  InheritSampleTime=on
  Mux : Mux  Inputs=2
  Out1 : Outport  VectorParamsAs1DForOutWhenUnconnected=off
  wires:
  Mux/1 -> MATLAB Function/2(set)
  Memory/1 -> Data Type Conversion/1
  In1/1 -> Mux/1
  MATLAB Function/1(y) -> Out1/1, Memory/1
  Data Type Conversion/1 -> MATLAB Function/1(yold)
  In2/1 -> Mux/2

== system Control_Logic_b_chk2/FF2 ==
  In1 : Inport
  In2 : Inport  Port=2
  Data Type Conversion : DataTypeConversion  OutDataTypeStr=boolean
  MATLAB Function : MATLAB Function  TreatAsAtomicUnit=on  SystemSampleTime=Sample_time
  Memory : Memory  InheritSampleTime=on
  Mux : Mux  Inputs=2
  Out1 : Outport  VectorParamsAs1DForOutWhenUnconnected=off
  wires:
  Mux/1 -> MATLAB Function/2(set)
  Memory/1 -> Data Type Conversion/1
  In1/1 -> Mux/1
  MATLAB Function/1(y) -> Out1/1, Memory/1
  Data Type Conversion/1 -> MATLAB Function/1(yold)
  In2/1 -> Mux/2

== system Control_Logic_b_chk2/FF3 ==
  In1 : Inport
  In2 : Inport  Port=2
  Data Type Conversion : DataTypeConversion  OutDataTypeStr=boolean
  MATLAB Function : MATLAB Function  TreatAsAtomicUnit=on  SystemSampleTime=Sample_time
  Memory : Memory  InheritSampleTime=on
  Mux : Mux  Inputs=2
  Out1 : Outport  VectorParamsAs1DForOutWhenUnconnected=off
  wires:
  Mux/1 -> MATLAB Function/2(set)
  Memory/1 -> Data Type Conversion/1
  In1/1 -> Mux/1
  MATLAB Function/1(y) -> Out1/1, Memory/1
  Data Type Conversion/1 -> MATLAB Function/1(yold)
  In2/1 -> Mux/2

== system Control_Logic_b_chk2/FF4 ==
  In1 : Inport
  In2 : Inport  Port=2
  Data Type Conversion : DataTypeConversion  OutDataTypeStr=boolean
  MATLAB Function : MATLAB Function  TreatAsAtomicUnit=on  SystemSampleTime=Sample_time
  Memory : Memory  InheritSampleTime=on
  Mux : Mux  Inputs=2
  Out1 : Outport  VectorParamsAs1DForOutWhenUnconnected=off
  wires:
  Mux/1 -> MATLAB Function/2(set)
  Memory/1 -> Data Type Conversion/1
  In1/1 -> Mux/1
  MATLAB Function/1(y) -> Out1/1, Memory/1
  Data Type Conversion/1 -> MATLAB Function/1(yold)
  In2/1 -> Mux/2

== system Control_Logic_b_chk2/First Order Lag1 ==
  In1 : Inport
  In2 : Inport  Port=2
  Discrete-Time Integrator : DiscreteIntegrator  InitialConditionSource=external  SampleTime=Sample_time  ICPrevOutput=DiscIntNeverNeededParam  ICPrevScaledInput=DiscIntNeverNeededParam
  Product : Product  Inputs=*/  SaturateOnIntegerOverflow=on  OutDataTypeStr=Inherit: Same as first input
  Sum : Sum  Inputs=|+-  SaturateOnIntegerOverflow=on
  Out1 : Outport  VectorParamsAs1DForOutWhenUnconnected=off
  wires:
  In1/1 -> Sum/1, Discrete-Time Integrator/2
  Discrete-Time Integrator/1 -> Out1/1, Sum/2
  Product/1 -> Discrete-Time Integrator/1
  Sum/1 -> Product/1
  In2/1 -> Product/2

== system Control_Logic_b_chk2/First Order Lag2 ==
  In1 : Inport
  In2 : Inport  Port=2
  Discrete-Time Integrator : DiscreteIntegrator  InitialConditionSource=external  SampleTime=Sample_time  ICPrevOutput=DiscIntNeverNeededParam  ICPrevScaledInput=DiscIntNeverNeededParam
  Product : Product  Inputs=*/  SaturateOnIntegerOverflow=on  OutDataTypeStr=Inherit: Same as first input
  Sum : Sum  Inputs=|+-  SaturateOnIntegerOverflow=on
  Out1 : Outport  VectorParamsAs1DForOutWhenUnconnected=off
  wires:
  In2/1 -> Product/2
  Sum/1 -> Product/1
  Product/1 -> Discrete-Time Integrator/1
  Discrete-Time Integrator/1 -> Sum/2, Out1/1
  In1/1 -> Discrete-Time Integrator/2, Sum/1

== system Control_Logic_b_chk2/First Order Lag5 ==
  In1 : Inport
  In2 : Inport  Port=2
  Discrete-Time Integrator : DiscreteIntegrator  InitialConditionSource=external  SampleTime=Sample_time  ICPrevOutput=DiscIntNeverNeededParam  ICPrevScaledInput=DiscIntNeverNeededParam
  Product : Product  Inputs=*/  SaturateOnIntegerOverflow=on  OutDataTypeStr=Inherit: Same as first input
  Sum : Sum  Inputs=|+-  SaturateOnIntegerOverflow=on
  Out1 : Outport  VectorParamsAs1DForOutWhenUnconnected=off
  wires:
  In2/1 -> Product/2
  Sum/1 -> Product/1
  Product/1 -> Discrete-Time Integrator/1
  Discrete-Time Integrator/1 -> Sum/2, Out1/1
  In1/1 -> Discrete-Time Integrator/2, Sum/1

== system Control_Logic_b_chk2/HLM ==
  In1 : Inport
  In2 : Inport  Port=2
  In3 : Inport  Port=3
  MATLAB Function : MATLAB Function  TreatAsAtomicUnit=on  SystemSampleTime=Sample_time
  Mux : Mux  Inputs=2
  Out1 : Outport  VectorParamsAs1DForOutWhenUnconnected=off
  wires:
  In3/1 -> Mux/2
  Mux/1 -> MATLAB Function/2(set)
  In1/1 -> MATLAB Function/1(u)
  MATLAB Function/1(y) -> Out1/1
  In2/1 -> Mux/1

== system Control_Logic_b_chk2/NOT ==
  In1 : Inport
  MATLAB Function : MATLAB Function  TreatAsAtomicUnit=on  SystemSampleTime=Sample_time
  Out1 : Outport  VectorParamsAs1DForOutWhenUnconnected=off
  wires:
  In1/1 -> MATLAB Function/1(u)
  MATLAB Function/1(y) -> Out1/1

== system Control_Logic_b_chk2/NOT1 ==
  In1 : Inport
  MATLAB Function : MATLAB Function  TreatAsAtomicUnit=on  SystemSampleTime=Sample_time
  Out1 : Outport  VectorParamsAs1DForOutWhenUnconnected=off
  wires:
  In1/1 -> MATLAB Function/1(u)
  MATLAB Function/1(y) -> Out1/1

== system Control_Logic_b_chk2/NOT2 ==
  In1 : Inport
  MATLAB Function : MATLAB Function  TreatAsAtomicUnit=on  SystemSampleTime=Sample_time
  Out1 : Outport  VectorParamsAs1DForOutWhenUnconnected=off
  wires:
  In1/1 -> MATLAB Function/1(u)
  MATLAB Function/1(y) -> Out1/1

== system Control_Logic_b_chk2/NOT3 ==
  In1 : Inport
  MATLAB Function : MATLAB Function  TreatAsAtomicUnit=on  SystemSampleTime=Sample_time
  Out1 : Outport  VectorParamsAs1DForOutWhenUnconnected=off
  wires:
  In1/1 -> MATLAB Function/1(u)
  MATLAB Function/1(y) -> Out1/1

== system Control_Logic_b_chk2/NOT4 ==
  In1 : Inport
  MATLAB Function : MATLAB Function  TreatAsAtomicUnit=on  SystemSampleTime=Sample_time
  Out1 : Outport  VectorParamsAs1DForOutWhenUnconnected=off
  wires:
  In1/1 -> MATLAB Function/1(u)
  MATLAB Function/1(y) -> Out1/1

== system Control_Logic_b_chk2/NOT5 ==
  In1 : Inport
  MATLAB Function : MATLAB Function  TreatAsAtomicUnit=on  SystemSampleTime=Sample_time
  Out1 : Outport  VectorParamsAs1DForOutWhenUnconnected=off
  wires:
  In1/1 -> MATLAB Function/1(u)
  MATLAB Function/1(y) -> Out1/1

== system Control_Logic_b_chk2/NOT6 ==
  In1 : Inport
  MATLAB Function : MATLAB Function  TreatAsAtomicUnit=on  SystemSampleTime=Sample_time
  Out1 : Outport  VectorParamsAs1DForOutWhenUnconnected=off
  wires:
  In1/1 -> MATLAB Function/1(u)
  MATLAB Function/1(y) -> Out1/1

== system Control_Logic_b_chk2/NOT7 ==
  In1 : Inport
  MATLAB Function : MATLAB Function  TreatAsAtomicUnit=on  SystemSampleTime=Sample_time
  Out1 : Outport  VectorParamsAs1DForOutWhenUnconnected=off
  wires:
  In1/1 -> MATLAB Function/1(u)
  MATLAB Function/1(y) -> Out1/1

== system Control_Logic_b_chk2/OFDLC ==
  In1 : Inport
  In2 : Inport  Port=2
  In3 : Inport  Port=3
  MATLAB Function : MATLAB Function  TreatAsAtomicUnit=on  SystemSampleTime=Sample_time
  Memory : Memory  InheritSampleTime=on
  Mux : Mux  Inputs=2
  Out1 : Outport  VectorParamsAs1DForOutWhenUnconnected=off
  wires:
  In3/1 -> Mux/1
  In2/1 -> MATLAB Function/2(set)
  Memory/1 -> Mux/2
  In1/1 -> MATLAB Function/1(ud)
  MATLAB Function/1(y) -> Out1/1
  MATLAB Function/2(w) -> Memory/1
  Mux/1 -> MATLAB Function/3(timc)

== system Control_Logic_b_chk2/OFDLC1 ==
  In1 : Inport
  In2 : Inport  Port=2
  In3 : Inport  Port=3
  MATLAB Function : MATLAB Function  TreatAsAtomicUnit=on  SystemSampleTime=Sample_time
  Memory : Memory  InheritSampleTime=on
  Mux : Mux  Inputs=2
  Out1 : Outport  VectorParamsAs1DForOutWhenUnconnected=off
  wires:
  In3/1 -> Mux/1
  In2/1 -> MATLAB Function/2(set)
  Memory/1 -> Mux/2
  In1/1 -> MATLAB Function/1(ud)
  MATLAB Function/1(y) -> Out1/1
  MATLAB Function/2(w) -> Memory/1
  Mux/1 -> MATLAB Function/3(timc)

== system Control_Logic_b_chk2/OFDLC2 ==
  In1 : Inport
  In2 : Inport  Port=2
  In3 : Inport  Port=3
  MATLAB Function : MATLAB Function  TreatAsAtomicUnit=on  SystemSampleTime=Sample_time
  Memory : Memory  InheritSampleTime=on
  Mux : Mux  Inputs=2
  Out1 : Outport  VectorParamsAs1DForOutWhenUnconnected=off
  wires:
  In3/1 -> Mux/1
  In2/1 -> MATLAB Function/2(set)
  Memory/1 -> Mux/2
  In1/1 -> MATLAB Function/1(ud)
  MATLAB Function/1(y) -> Out1/1
  MATLAB Function/2(w) -> Memory/1
  Mux/1 -> MATLAB Function/3(timc)

== system Control_Logic_b_chk2/OFDLC3 ==
  In1 : Inport
  In2 : Inport  Port=2
  In3 : Inport  Port=3
  MATLAB Function : MATLAB Function  TreatAsAtomicUnit=on  SystemSampleTime=Sample_time
  Memory : Memory  InheritSampleTime=on
  Mux : Mux  Inputs=2
  Out1 : Outport  VectorParamsAs1DForOutWhenUnconnected=off
  wires:
  In3/1 -> Mux/1
  In2/1 -> MATLAB Function/2(set)
  Memory/1 -> Mux/2
  In1/1 -> MATLAB Function/1(ud)
  MATLAB Function/1(y) -> Out1/1
  MATLAB Function/2(w) -> Memory/1
  Mux/1 -> MATLAB Function/3(timc)

== system Control_Logic_b_chk2/ONDLC ==
  In1 : Inport
  In2 : Inport  Port=2
  In3 : Inport  Port=3
  MATLAB Function : MATLAB Function  TreatAsAtomicUnit=on  SystemSampleTime=Sample_time
  Memory : Memory  InheritSampleTime=on
  Mux : Mux  Inputs=2
  Out1 : Outport  VectorParamsAs1DForOutWhenUnconnected=off
  wires:
  In3/1 -> Mux/1
  Memory/1 -> Mux/2
  In1/1 -> MATLAB Function/1(ud)
  MATLAB Function/1(y) -> Out1/1
  Mux/1 -> MATLAB Function/3(timc)
  In2/1 -> MATLAB Function/2(set)
  MATLAB Function/2(w) -> Memory/1

== system Control_Logic_b_chk2/ONDLC1 ==
  In1 : Inport
  In2 : Inport  Port=2
  In3 : Inport  Port=3
  MATLAB Function : MATLAB Function  TreatAsAtomicUnit=on  SystemSampleTime=Sample_time
  Memory : Memory  InheritSampleTime=on
  Mux : Mux  Inputs=2
  Out1 : Outport  VectorParamsAs1DForOutWhenUnconnected=off
  wires:
  In3/1 -> Mux/1
  Memory/1 -> Mux/2
  In1/1 -> MATLAB Function/1(ud)
  MATLAB Function/1(y) -> Out1/1
  Mux/1 -> MATLAB Function/3(timc)
  In2/1 -> MATLAB Function/2(set)
  MATLAB Function/2(w) -> Memory/1

== system Control_Logic_b_chk2/ONDLC2 ==
  In1 : Inport
  In2 : Inport  Port=2
  In3 : Inport  Port=3
  MATLAB Function : MATLAB Function  TreatAsAtomicUnit=on  SystemSampleTime=Sample_time
  Memory : Memory  InheritSampleTime=on
  Mux : Mux  Inputs=2
  Out1 : Outport  VectorParamsAs1DForOutWhenUnconnected=off
  wires:
  In3/1 -> Mux/1
  Memory/1 -> Mux/2
  In1/1 -> MATLAB Function/1(ud)
  MATLAB Function/1(y) -> Out1/1
  Mux/1 -> MATLAB Function/3(timc)
  In2/1 -> MATLAB Function/2(set)
  MATLAB Function/2(w) -> Memory/1

== system Control_Logic_b_chk2/ONDLC3 ==
  In1 : Inport
  In2 : Inport  Port=2
  In3 : Inport  Port=3
  MATLAB Function : MATLAB Function  TreatAsAtomicUnit=on  SystemSampleTime=Sample_time
  Memory : Memory  InheritSampleTime=on
  Mux : Mux  Inputs=2
  Out1 : Outport  VectorParamsAs1DForOutWhenUnconnected=off
  wires:
  In3/1 -> Mux/1
  Memory/1 -> Mux/2
  In1/1 -> MATLAB Function/1(ud)
  MATLAB Function/1(y) -> Out1/1
  Mux/1 -> MATLAB Function/3(timc)
  In2/1 -> MATLAB Function/2(set)
  MATLAB Function/2(w) -> Memory/1

== system Control_Logic_b_chk2/OR ==
  In1 : Inport
  In2 : Inport  Port=2
  MATLAB Function : MATLAB Function  TreatAsAtomicUnit=on  SystemSampleTime=Sample_time
  Mux : Mux  Inputs=2
  Out1 : Outport  VectorParamsAs1DForOutWhenUnconnected=off
  wires:
  Mux/1 -> MATLAB Function/1(u)
  MATLAB Function/1(y) -> Out1/1
  In1/1 -> Mux/1
  In2/1 -> Mux/2

== system Control_Logic_b_chk2/OR1 ==
  In1 : Inport
  In2 : Inport  Port=2
  MATLAB Function : MATLAB Function  TreatAsAtomicUnit=on  SystemSampleTime=Sample_time
  Mux : Mux  Inputs=2
  Out1 : Outport  VectorParamsAs1DForOutWhenUnconnected=off
  wires:
  Mux/1 -> MATLAB Function/1(u)
  MATLAB Function/1(y) -> Out1/1
  In1/1 -> Mux/1
  In2/1 -> Mux/2

== system Control_Logic_b_chk2/OR2 ==
  In1 : Inport
  In2 : Inport  Port=2
  MATLAB Function : MATLAB Function  TreatAsAtomicUnit=on  SystemSampleTime=Sample_time
  Mux : Mux  Inputs=2
  Out1 : Outport  VectorParamsAs1DForOutWhenUnconnected=off
  wires:
  Mux/1 -> MATLAB Function/1(u)
  MATLAB Function/1(y) -> Out1/1
  In1/1 -> Mux/1
  In2/1 -> Mux/2

== system Control_Logic_b_chk2/OR3L ==
  In1 : Inport
  In2 : Inport  Port=2
  In3 : Inport  Port=3
  MATLAB Function : MATLAB Function  TreatAsAtomicUnit=on  SystemSampleTime=Sample_time
  Mux : Mux  Inputs=3
  Out1 : Outport  VectorParamsAs1DForOutWhenUnconnected=off
  wires:
  Mux/1 -> MATLAB Function/1(u)
  In3/1 -> Mux/3
  In1/1 -> Mux/1
  MATLAB Function/1(y) -> Out1/1
  In2/1 -> Mux/2

== system Control_Logic_b_chk2/OR3L1 ==
  In1 : Inport
  In2 : Inport  Port=2
  In3 : Inport  Port=3
  MATLAB Function : MATLAB Function  TreatAsAtomicUnit=on  SystemSampleTime=Sample_time
  Mux : Mux  Inputs=3
  Out1 : Outport  VectorParamsAs1DForOutWhenUnconnected=off
  wires:
  Mux/1 -> MATLAB Function/1(u)
  In3/1 -> Mux/3
  In1/1 -> Mux/1
  MATLAB Function/1(y) -> Out1/1
  In2/1 -> Mux/2

== system Control_Logic_b_chk2/OR3L2 ==
  In1 : Inport
  In2 : Inport  Port=2
  In3 : Inport  Port=3
  MATLAB Function : MATLAB Function  TreatAsAtomicUnit=on  SystemSampleTime=Sample_time
  Mux : Mux  Inputs=3
  Out1 : Outport  VectorParamsAs1DForOutWhenUnconnected=off
  wires:
  Mux/1 -> MATLAB Function/1(u)
  In3/1 -> Mux/3
  In1/1 -> Mux/1
  MATLAB Function/1(y) -> Out1/1
  In2/1 -> Mux/2

== system Control_Logic_b_chk2/OR3L3 ==
  In1 : Inport
  In2 : Inport  Port=2
  In3 : Inport  Port=3
  MATLAB Function : MATLAB Function  TreatAsAtomicUnit=on  SystemSampleTime=Sample_time
  Mux : Mux  Inputs=3
  Out1 : Outport  VectorParamsAs1DForOutWhenUnconnected=off
  wires:
  Mux/1 -> MATLAB Function/1(u)
  In3/1 -> Mux/3
  In1/1 -> Mux/1
  MATLAB Function/1(y) -> Out1/1
  In2/1 -> Mux/2

== system Control_Logic_b_chk2/OR3L4 ==
  In1 : Inport
  In2 : Inport  Port=2
  In3 : Inport  Port=3
  MATLAB Function : MATLAB Function  TreatAsAtomicUnit=on  SystemSampleTime=Sample_time
  Mux : Mux  Inputs=3
  Out1 : Outport  VectorParamsAs1DForOutWhenUnconnected=off
  wires:
  Mux/1 -> MATLAB Function/1(u)
  In3/1 -> Mux/3
  In1/1 -> Mux/1
  MATLAB Function/1(y) -> Out1/1
  In2/1 -> Mux/2

== system Control_Logic_b_chk2/OR3L5 ==
  In1 : Inport
  In2 : Inport  Port=2
  In3 : Inport  Port=3
  MATLAB Function : MATLAB Function  TreatAsAtomicUnit=on  SystemSampleTime=Sample_time
  Mux : Mux  Inputs=3
  Out1 : Outport  VectorParamsAs1DForOutWhenUnconnected=off
  wires:
  Mux/1 -> MATLAB Function/1(u)
  In3/1 -> Mux/3
  In1/1 -> Mux/1
  MATLAB Function/1(y) -> Out1/1
  In2/1 -> Mux/2

== system Control_Logic_b_chk2/OR3L6 ==
  In1 : Inport
  In2 : Inport  Port=2
  In3 : Inport  Port=3
  MATLAB Function : MATLAB Function  TreatAsAtomicUnit=on  SystemSampleTime=Sample_time
  Mux : Mux  Inputs=3
  Out1 : Outport  VectorParamsAs1DForOutWhenUnconnected=off
  wires:
  Mux/1 -> MATLAB Function/1(u)
  In3/1 -> Mux/3
  In1/1 -> Mux/1
  MATLAB Function/1(y) -> Out1/1
  In2/1 -> Mux/2

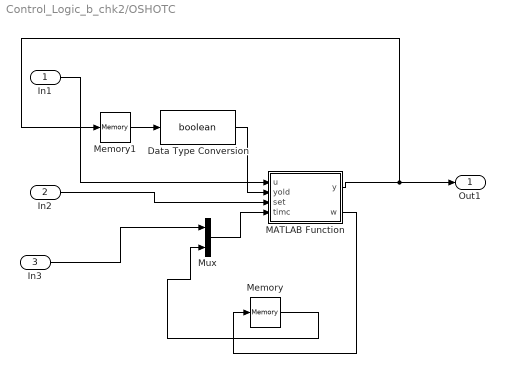
== system Control_Logic_b_chk2/OSHOTC ==
  In1 : Inport
  In2 : Inport  Port=2
  In3 : Inport  Port=3
  Data Type Conversion : DataTypeConversion  OutDataTypeStr=boolean
  MATLAB Function : MATLAB Function  TreatAsAtomicUnit=on  SystemSampleTime=Sample_time
  Memory : Memory  InheritSampleTime=on
  Memory1 : Memory  InheritSampleTime=on  LinearizeAsDelay=on
  Mux : Mux  Inputs=2
  Out1 : Outport  VectorParamsAs1DForOutWhenUnconnected=off
  wires:
  Memory/1 -> Mux/2
  MATLAB Function/1(y) -> Out1/1, Memory1/1
  In2/1 -> MATLAB Function/3(set)
  Mux/1 -> MATLAB Function/4(timc)
  In1/1 -> MATLAB Function/1(u)
  Memory1/1 -> Data Type Conversion/1
  Data Type Conversion/1 -> MATLAB Function/2(yold)
  MATLAB Function/2(w) -> Memory/1
  In3/1 -> Mux/1

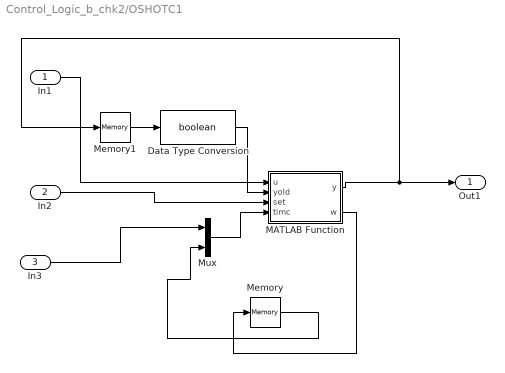
== system Control_Logic_b_chk2/OSHOTC1 ==
  In1 : Inport
  In2 : Inport  Port=2
  In3 : Inport  Port=3
  Data Type Conversion : DataTypeConversion  OutDataTypeStr=boolean
  MATLAB Function : MATLAB Function  TreatAsAtomicUnit=on  SystemSampleTime=Sample_time
  Memory : Memory  InheritSampleTime=on
  Memory1 : Memory  InheritSampleTime=on  LinearizeAsDelay=on
  Mux : Mux  Inputs=2
  Out1 : Outport  VectorParamsAs1DForOutWhenUnconnected=off
  wires:
  Memory/1 -> Mux/2
  MATLAB Function/1(y) -> Out1/1, Memory1/1
  In2/1 -> MATLAB Function/3(set)
  Mux/1 -> MATLAB Function/4(timc)
  In1/1 -> MATLAB Function/1(u)
  Memory1/1 -> Data Type Conversion/1
  Data Type Conversion/1 -> MATLAB Function/2(yold)
  MATLAB Function/2(w) -> Memory/1
  In3/1 -> Mux/1

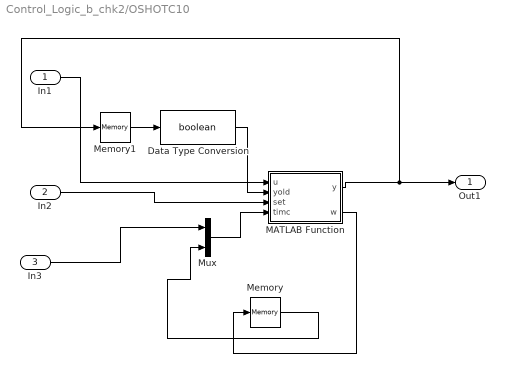
== system Control_Logic_b_chk2/OSHOTC10 ==
  In1 : Inport
  In2 : Inport  Port=2
  In3 : Inport  Port=3
  Data Type Conversion : DataTypeConversion  OutDataTypeStr=boolean
  MATLAB Function : MATLAB Function  TreatAsAtomicUnit=on  SystemSampleTime=Sample_time
  Memory : Memory  InheritSampleTime=on
  Memory1 : Memory  InheritSampleTime=on  LinearizeAsDelay=on
  Mux : Mux  Inputs=2
  Out1 : Outport  VectorParamsAs1DForOutWhenUnconnected=off
  wires:
  Memory/1 -> Mux/2
  MATLAB Function/1(y) -> Out1/1, Memory1/1
  In2/1 -> MATLAB Function/3(set)
  Mux/1 -> MATLAB Function/4(timc)
  In1/1 -> MATLAB Function/1(u)
  Memory1/1 -> Data Type Conversion/1
  Data Type Conversion/1 -> MATLAB Function/2(yold)
  MATLAB Function/2(w) -> Memory/1
  In3/1 -> Mux/1

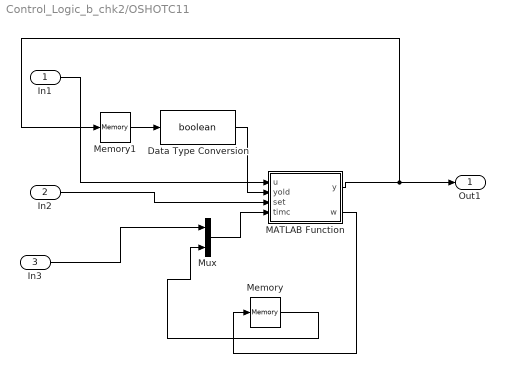
== system Control_Logic_b_chk2/OSHOTC11 ==
  In1 : Inport
  In2 : Inport  Port=2
  In3 : Inport  Port=3
  Data Type Conversion : DataTypeConversion  OutDataTypeStr=boolean
  MATLAB Function : MATLAB Function  TreatAsAtomicUnit=on  SystemSampleTime=Sample_time
  Memory : Memory  InheritSampleTime=on
  Memory1 : Memory  InheritSampleTime=on  LinearizeAsDelay=on
  Mux : Mux  Inputs=2
  Out1 : Outport  VectorParamsAs1DForOutWhenUnconnected=off
  wires:
  Memory/1 -> Mux/2
  MATLAB Function/1(y) -> Out1/1, Memory1/1
  In2/1 -> MATLAB Function/3(set)
  Mux/1 -> MATLAB Function/4(timc)
  In1/1 -> MATLAB Function/1(u)
  Memory1/1 -> Data Type Conversion/1
  Data Type Conversion/1 -> MATLAB Function/2(yold)
  MATLAB Function/2(w) -> Memory/1
  In3/1 -> Mux/1

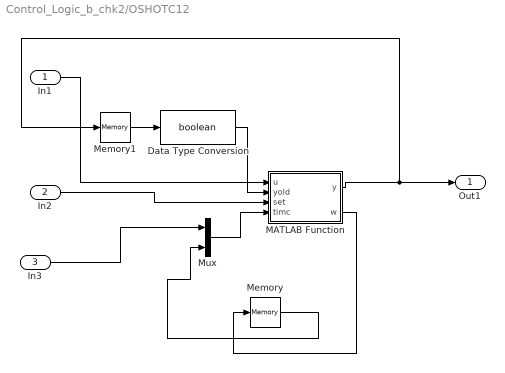
== system Control_Logic_b_chk2/OSHOTC12 ==
  In1 : Inport
  In2 : Inport  Port=2
  In3 : Inport  Port=3
  Data Type Conversion : DataTypeConversion  OutDataTypeStr=boolean
  MATLAB Function : MATLAB Function  TreatAsAtomicUnit=on  SystemSampleTime=Sample_time
  Memory : Memory  InheritSampleTime=on
  Memory1 : Memory  InheritSampleTime=on  LinearizeAsDelay=on
  Mux : Mux  Inputs=2
  Out1 : Outport  VectorParamsAs1DForOutWhenUnconnected=off
  wires:
  Memory/1 -> Mux/2
  MATLAB Function/1(y) -> Out1/1, Memory1/1
  In2/1 -> MATLAB Function/3(set)
  Mux/1 -> MATLAB Function/4(timc)
  In1/1 -> MATLAB Function/1(u)
  Memory1/1 -> Data Type Conversion/1
  Data Type Conversion/1 -> MATLAB Function/2(yold)
  MATLAB Function/2(w) -> Memory/1
  In3/1 -> Mux/1

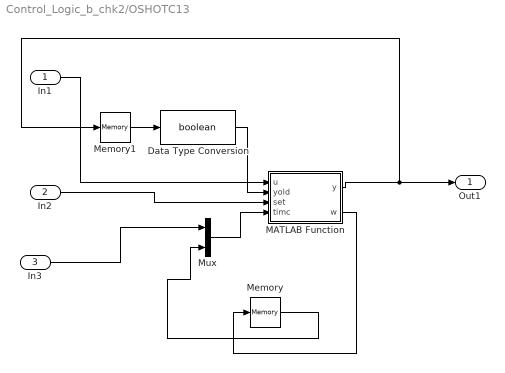
== system Control_Logic_b_chk2/OSHOTC13 ==
  In1 : Inport
  In2 : Inport  Port=2
  In3 : Inport  Port=3
  Data Type Conversion : DataTypeConversion  OutDataTypeStr=boolean
  MATLAB Function : MATLAB Function  TreatAsAtomicUnit=on  SystemSampleTime=Sample_time
  Memory : Memory  InheritSampleTime=on
  Memory1 : Memory  InheritSampleTime=on  LinearizeAsDelay=on
  Mux : Mux  Inputs=2
  Out1 : Outport  VectorParamsAs1DForOutWhenUnconnected=off
  wires:
  Memory/1 -> Mux/2
  MATLAB Function/1(y) -> Out1/1, Memory1/1
  In2/1 -> MATLAB Function/3(set)
  Mux/1 -> MATLAB Function/4(timc)
  In1/1 -> MATLAB Function/1(u)
  Memory1/1 -> Data Type Conversion/1
  Data Type Conversion/1 -> MATLAB Function/2(yold)
  MATLAB Function/2(w) -> Memory/1
  In3/1 -> Mux/1

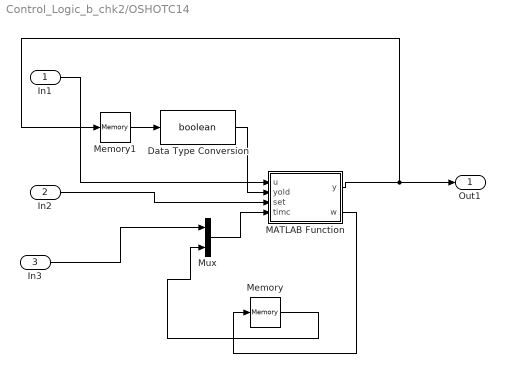
== system Control_Logic_b_chk2/OSHOTC14 ==
  In1 : Inport
  In2 : Inport  Port=2
  In3 : Inport  Port=3
  Data Type Conversion : DataTypeConversion  OutDataTypeStr=boolean
  MATLAB Function : MATLAB Function  TreatAsAtomicUnit=on  SystemSampleTime=Sample_time
  Memory : Memory  InheritSampleTime=on
  Memory1 : Memory  InheritSampleTime=on  LinearizeAsDelay=on
  Mux : Mux  Inputs=2
  Out1 : Outport  VectorParamsAs1DForOutWhenUnconnected=off
  wires:
  Memory/1 -> Mux/2
  MATLAB Function/1(y) -> Out1/1, Memory1/1
  In2/1 -> MATLAB Function/3(set)
  Mux/1 -> MATLAB Function/4(timc)
  In1/1 -> MATLAB Function/1(u)
  Memory1/1 -> Data Type Conversion/1
  Data Type Conversion/1 -> MATLAB Function/2(yold)
  MATLAB Function/2(w) -> Memory/1
  In3/1 -> Mux/1

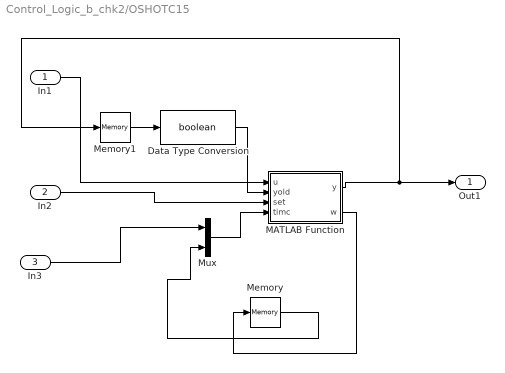
== system Control_Logic_b_chk2/OSHOTC15 ==
  In1 : Inport
  In2 : Inport  Port=2
  In3 : Inport  Port=3
  Data Type Conversion : DataTypeConversion  OutDataTypeStr=boolean
  MATLAB Function : MATLAB Function  TreatAsAtomicUnit=on  SystemSampleTime=Sample_time
  Memory : Memory  InheritSampleTime=on
  Memory1 : Memory  InheritSampleTime=on  LinearizeAsDelay=on
  Mux : Mux  Inputs=2
  Out1 : Outport  VectorParamsAs1DForOutWhenUnconnected=off
  wires:
  Memory/1 -> Mux/2
  MATLAB Function/1(y) -> Out1/1, Memory1/1
  In2/1 -> MATLAB Function/3(set)
  Mux/1 -> MATLAB Function/4(timc)
  In1/1 -> MATLAB Function/1(u)
  Memory1/1 -> Data Type Conversion/1
  Data Type Conversion/1 -> MATLAB Function/2(yold)
  MATLAB Function/2(w) -> Memory/1
  In3/1 -> Mux/1

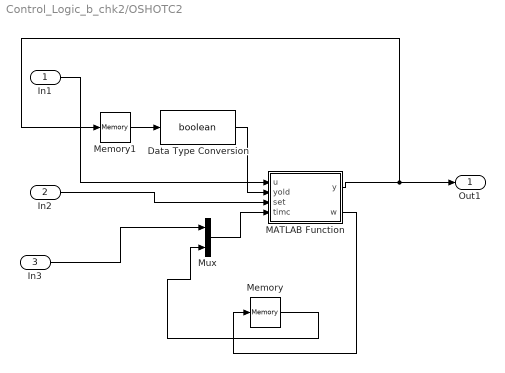
== system Control_Logic_b_chk2/OSHOTC2 ==
  In1 : Inport
  In2 : Inport  Port=2
  In3 : Inport  Port=3
  Data Type Conversion : DataTypeConversion  OutDataTypeStr=boolean
  MATLAB Function : MATLAB Function  TreatAsAtomicUnit=on  SystemSampleTime=Sample_time
  Memory : Memory  InheritSampleTime=on
  Memory1 : Memory  InheritSampleTime=on  LinearizeAsDelay=on
  Mux : Mux  Inputs=2
  Out1 : Outport  VectorParamsAs1DForOutWhenUnconnected=off
  wires:
  Memory/1 -> Mux/2
  MATLAB Function/1(y) -> Out1/1, Memory1/1
  In2/1 -> MATLAB Function/3(set)
  Mux/1 -> MATLAB Function/4(timc)
  In1/1 -> MATLAB Function/1(u)
  Memory1/1 -> Data Type Conversion/1
  Data Type Conversion/1 -> MATLAB Function/2(yold)
  MATLAB Function/2(w) -> Memory/1
  In3/1 -> Mux/1

== system Control_Logic_b_chk2/OSHOTC3 ==
  In1 : Inport
  In2 : Inport  Port=2
  In3 : Inport  Port=3
  Data Type Conversion : DataTypeConversion  OutDataTypeStr=boolean
  MATLAB Function : MATLAB Function  TreatAsAtomicUnit=on  SystemSampleTime=Sample_time
  Memory : Memory  InheritSampleTime=on
  Memory1 : Memory  InheritSampleTime=on  LinearizeAsDelay=on
  Mux : Mux  Inputs=2
  Out1 : Outport  VectorParamsAs1DForOutWhenUnconnected=off
  wires:
  Memory/1 -> Mux/2
  MATLAB Function/1(y) -> Out1/1, Memory1/1
  In2/1 -> MATLAB Function/3(set)
  Mux/1 -> MATLAB Function/4(timc)
  In1/1 -> MATLAB Function/1(u)
  Memory1/1 -> Data Type Conversion/1
  Data Type Conversion/1 -> MATLAB Function/2(yold)
  MATLAB Function/2(w) -> Memory/1
  In3/1 -> Mux/1

== system Control_Logic_b_chk2/OSHOTC4 ==
  In1 : Inport
  In2 : Inport  Port=2
  In3 : Inport  Port=3
  Data Type Conversion : DataTypeConversion  OutDataTypeStr=boolean
  MATLAB Function : MATLAB Function  TreatAsAtomicUnit=on  SystemSampleTime=Sample_time
  Memory : Memory  InheritSampleTime=on
  Memory1 : Memory  InheritSampleTime=on  LinearizeAsDelay=on
  Mux : Mux  Inputs=2
  Out1 : Outport  VectorParamsAs1DForOutWhenUnconnected=off
  wires:
  Memory/1 -> Mux/2
  MATLAB Function/1(y) -> Out1/1, Memory1/1
  In2/1 -> MATLAB Function/3(set)
  Mux/1 -> MATLAB Function/4(timc)
  In1/1 -> MATLAB Function/1(u)
  Memory1/1 -> Data Type Conversion/1
  Data Type Conversion/1 -> MATLAB Function/2(yold)
  MATLAB Function/2(w) -> Memory/1
  In3/1 -> Mux/1
